simulink library "HighFrequencyNoiseEstimatorCoh"  (R2022b)
settings: Solver=VariableStepAuto  StartTime=0.0  StopTime=10.0  RelTol=1e-3
values from neighbouring files (symbols this model uses):
  NumAAChannels = NumHFRefChannels + 1    [HighFrequencyNoiseEstimatorCohMask.m]
  NumHFRefChannels = NumHFRefLPF + NumHFRefBPF    [HighFrequencyNoiseEstimatorCohMask.m]
undefined symbols (not defined in the file or in its folder): magnitude, Row
libraries: TuneVar x46, TOP x12, StateVar x10, FeaturePath x7, HandyTextFile x4, RfftLib x2, dspmathops x2, dspobslib x2, SpeedBoundsNoiseSlew x2, PooliirLib x2, TSP x1, dspsrcs4 x1
(part 1 of 2)
settings Model: Creator=zs14328  LastModifiedBy=sc48041
settings SolverCC: AlgebraicLoopSolver=TrustRegion
settings DataIOCC: ReturnWorkspaceOutputs=off
settings DebuggingCC: UnconnectedInputMsg=warning  UnconnectedOutputMsg=warning  UnconnectedLineMsg=warning  SFMachineParentedDataDiag=warning  ArithmeticOperatorsInVariantConditions=warning
settings ModelReferenceCC: EnableRefExpFcnMdlSchedulingChecks=on
settings SFSimCC: CustomCodeUndefinedFunction=UseInterfaceOnly

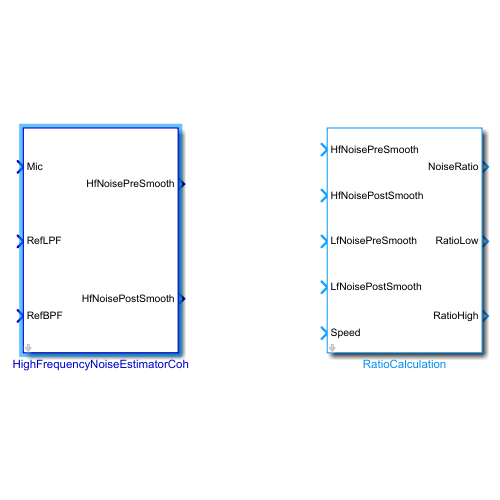
[thumbnail: Simulink's stored preview of the top-level diagram]
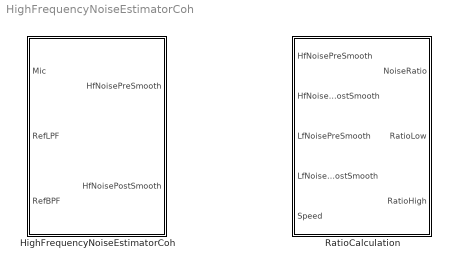
== system HighFrequencyNoiseEstimatorCoh ==
  HighFrequencyNoiseEstimatorCoh : Subsystem  mask(AudioPilot - High-Frequency Noise Estimator){FeatureName=HfNoise, NumHFRefLPF=4, NumHFRefBPF=3, Config=[], TriggerInit=0}
      mask prompts: FeatureName "Feature Name:"; NumHFRefLPF "Number of "High-Pass" Reference Channels"; NumHFRefBPF "Number of "Full-Band" Reference Channels"; Config "HighFrequencyNoiseEstimatorCohConfig"
      mask help: This block implements the high-frequency noise estimator based on the multi-coherence method.
      mask init:
      | blkh = gcbh;
      | 
      | Config = BTConfig.Assert(blkh,Config);
      | Config.Validate();
      | 
      | % Matlab Function Parameters
      | FrameSize = Config.FrameSize;
      | SampleRate = Config.SampleRateHz;
      | HFDecRate = Config.DecRateHz;
      | HFDecRate2 = Config.CoherenceDecRateHz;
      | HFDecRate3 = Config.CoherenceDecRate2Hz;   
      | 
      | % Constants
      | 
      | EmptyStftInput = zeros((FrameSize/Config.DecimationFactor),1);
      |           
      | % Create the PoolIIR Coefficients and Parameters           
      | [AA, BPLP, NumAAChannels, NumHFRefChannels] ...
      |     = HighFrequencyNoiseEstimatorCohMask.FormFilterCoef ...
      |                 (blkh,Config,NumHFRefLPF,NumHFRefBPF);
      | 
      | % Configure Model according to Mask & Config Parameters            
      | HighFrequencyNoiseEstimatorCohMask.ConfigureModel ...
      |                 (blkh,NumHFRefLPF,NumHFRefBPF,Config);
      | 
      | BTConfig.InitSetFeatureIfPresent(blkh,'FeatureName');
      mask Help:
      | Arguments for this block:
      | 
      | Design Time Configuration
      | 
      | Feature Name -
      | The Feature Name can be specified unless a BTC instance is used, in which case, the instance name will be used as Feature Name.
      | 
      | Number of "High-Pass"Reference Channels -
      | These are the reference channels from Medusa that have already been high-passed, such as  Limp, Rimp etc.  These channels will then undergo low-pass filtering only.
      | 
      | Number of "Full-Band" Reference Channels -
      | These are the reference channels from Medusa that are essentially full-band, such as LStreb, RStreb etc.  These channels will then undergo band-pass filtering.
      | 
      | Build Time Configuration -
      | The block can be configured using a object of class, HighFrequencyNoiseEstimatorCohConfig.
      mask TypeOptions FeatureName: FeaturePath/FeatureName
      mask Callback Config: BTConfig.CallbackHideIfPresent(gcbh,{'FeatureName'});
      mask Callback TriggerInit: HighFrequencyNoiseEstimatorCohMask.TriggerInitCallBack(gcbh);
      mask DialogControl DTCTitle Prompt: <b>Design Time Configuration</b>
      mask DialogControl BTCTitle Prompt: <b>Build Time Configuration</b>
  RatioCalculation : Subsystem  mask(AudioPilot - Noise Ratio Calculation){FeatureName=Ratio, Config=[]}
      mask prompts: FeatureName "Feature Name:"; Config "RatioCalculationConfig"
      mask help: This block handles the computation, smoothing and impulse rejection of the noise ratio.
      mask init:
      | blkh = gcbh;
      | 
      | Config = BTConfig.Assert(blkh,Config);
      | Config.Validate();
      | 
      | SampleRate = Config.SampleRateHz;
      | HFDecRate = Config.DecRateHz;
      |  
      | BTConfig.InitSetFeatureIfPresent(blkh,'FeatureName');
      mask Help:
      | This block handles the computation, smoothing and impulse rejection of the noise ratio.
      | 
      | Arguments for this block:
      | 
      | Design Time Configuration
      | The Feature Name can be specified unless a BTC instance is used, in which case, the instance name will be used as Feature Name.
      | 
      | Build Time Configuration
      | The block can be configured using a object of class, RatioCalculationConfig.
      mask TypeOptions FeatureName: FeaturePath/FeatureName
      mask Callback Config: BTConfig.CallbackHideIfPresent(gcbh,{'FeatureName'});
      mask DialogControl DTCTitle Prompt: <b>Design Time Configuration </b>
      mask DialogControl BTCTitle Prompt: <b>Build Time Configuration </b>
      mask DialogControl Config Tooltip: The configuration has to be an object of the class, RatioCalculationConfig.

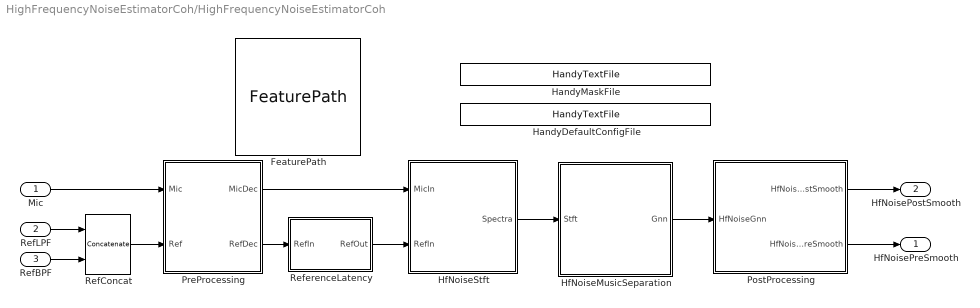
== system HighFrequencyNoiseEstimatorCoh/HighFrequencyNoiseEstimatorCoh ==
  Mic : Inport
  RefLPF : Inport  Port=2  PortDimensions=[FrameSize NumHFRefLPF]
  RefBPF : Inport  Port=3  PortDimensions=[FrameSize NumHFRefBPF]
  FeaturePath : FeaturePath/FeaturePath  FeatureName=HfNoise  IsGroup=off  GroupNumber=-1  IsModule=off  TriggerInit=[360 -186 485 -69]
      settings: SourceProductName=Bose Talaria
  HandyDefaultConfigFile : HandyTextFile/HandyTextFile  TemplateSource=Config  FileSuffix=Init  OpenDialogOnLoad=off  UseThisBlockName=off  AddGrandParentNamePrefix=off  TheDefaultText=|  ShowInLibBrowser=on
      | % $(FILENAME) Setup model parameters for each "Init" callback (e.g. update diagram)
      | sample_rate_in_hertz = 44100;
      | frame_size = 32;
      | sysin_channel_count = 2;
      settings: SourceProductName=Bose Talaria
  HandyMaskFile : HandyTextFile/HandyTextFile  TemplateSource=<dialog fields>  FileSuffix=Mask  OpenDialogOnLoad=off  UseThisBlockName=off  AddGrandParentNamePrefix=off  TheDefaultText=|  ShowInLibBrowser=on
      | % $(FILENAME) Setup model parameters for each "Init" callback (e.g. update diagram)
      | sample_rate_in_hertz = 44100;
      | frame_size = 32;
      | sysin_channel_count = 2;
      settings: SourceProductName=Bose Talaria
  "HfNoiseMusicSeparation " : Subsystem
  HfNoiseStft : Subsystem  Variant=on  VariantControlMode=label  LabelModeActiveChoice=EvenNumChannels
  PostProcessing : Subsystem
  PreProcessing : Subsystem
  RefConcat : Concatenate  Mode=Multidimensional array  ConcatenateDimension=2
  ReferenceLatency : Subsystem
  HfNoisePreSmooth : Outport  VectorParamsAs1DForOutWhenUnconnected=off
  HfNoisePostSmooth : Outport  Port=2  VectorParamsAs1DForOutWhenUnconnected=off
  wires:
  "HfNoiseMusicSeparation "/1(Gnn) -> PostProcessing/1(HfNoiseGnn)
  PreProcessing/2(RefDec) -> ReferenceLatency/1(RefIn)
  PreProcessing/1(MicDec) -> HfNoiseStft/1(MicIn)
  PostProcessing/2(HfNoisePreSmooth) -> HfNoisePreSmooth/1
  PostProcessing/1(HfNoisePostSmooth) -> HfNoisePostSmooth/1
  Mic/1 -> PreProcessing/1(Mic)
  HfNoiseStft/1(Spectra) -> "HfNoiseMusicSeparation "/1(Stft)
  ReferenceLatency/1(RefOut) -> HfNoiseStft/2(RefIn)
  RefConcat/1 -> PreProcessing/2(Ref)
  RefLPF/1 -> RefConcat/1
  RefBPF/1 -> RefConcat/2

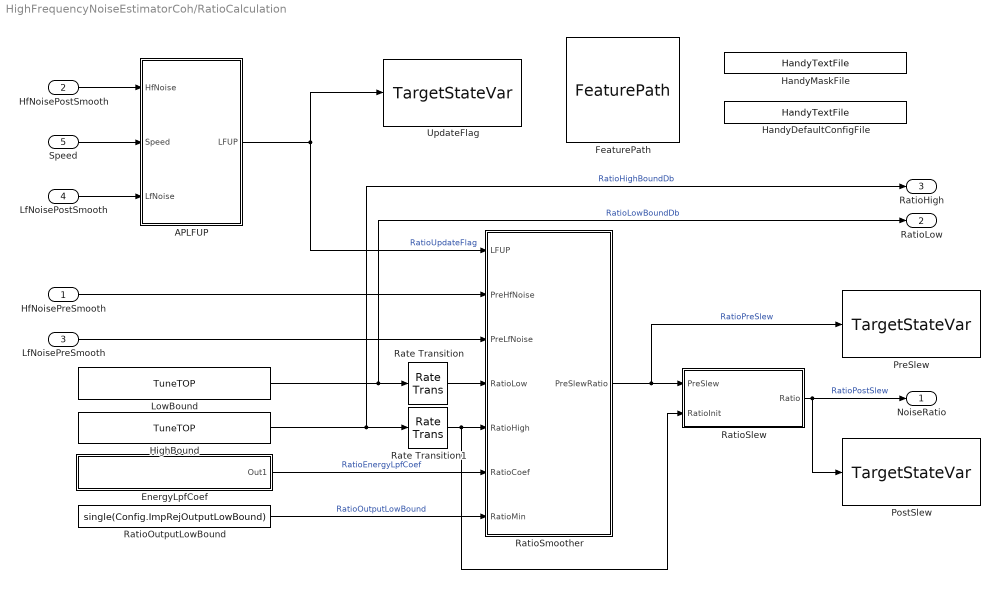
== system HighFrequencyNoiseEstimatorCoh/RatioCalculation ==
  HfNoisePreSmooth : Inport  SampleTime=Config.DecSampleTimeSec
  HfNoisePostSmooth : Inport  Port=2  SampleTime=Config.DecSampleTimeSec
  LfNoisePreSmooth : Inport  Port=3  SampleTime=Config.DecSampleTimeSec
  LfNoisePostSmooth : Inport  Port=4  SampleTime=Config.DecSampleTimeSec
  Speed : Inport  Port=5  SampleTime=Config.DecSampleTimeSec
  APLFUP : Subsystem
  EnergyLpfCoef : Subsystem
  FeaturePath : FeaturePath/FeaturePath  FeatureName=Ratio  IsGroup=off  GroupNumber=-1  IsModule=off  TriggerInit=[735 -166 850 -59]
      settings: SourceProductName=Bose Talaria
  HandyDefaultConfigFile : HandyTextFile/HandyTextFile  TemplateSource=Config  FileSuffix=Init  OpenDialogOnLoad=off  UseThisBlockName=off  TheDefaultText=|  ShowInLibBrowser=on
      | % $(FILENAME) Setup model parameters for each "Init" callback (e.g. update diagram)
      | sample_rate_in_hertz = 44100;
      | frame_size = 32;
      | sysin_channel_count = 2;
      settings: SourceProductName=Bose Talaria
  HandyMaskFile : HandyTextFile/HandyTextFile  TemplateSource=Mask  FileSuffix=Init  OpenDialogOnLoad=off  UseThisBlockName=off  TheDefaultText=|  ShowInLibBrowser=on
      | % $(FILENAME) Setup model parameters for each "Init" callback (e.g. update diagram)
      | sample_rate_in_hertz = 44100;
      | frame_size = 32;
      | sysin_channel_count = 2;
      settings: SourceProductName=Bose Talaria
  HighBound : TuneVar/TuneTOP  TriggerInit=[240 214 435 246]  TopName=HighBoundDb  TuneName=HighBoundDb  DataType=single  TunabilityNumber=1  MinValue=[]  MaxValue=[]  BankNumber=0  PreOverlay=false  PostOverlay=false  UseSameName=on  MaskValue=Config.HighBoundDb
      settings: SourceProductName=Bose Talaria
  LowBound : TuneVar/TuneTOP  TriggerInit=[240 169 435 201]  TopName=LowBoundDb  TuneName=LowBoundDb  DataType=single  TunabilityNumber=1  MinValue=[]  MaxValue=[]  BankNumber=0  PreOverlay=false  PostOverlay=false  UseSameName=on  MaskValue=Config.LowBoundDb
      settings: SourceProductName=Bose Talaria
  PostSlew : StateVar/TargetStateVar  TriggerInit=[1015 241 1155 309]  TspName=PostSlew  StateName=PostSlew  UseSameName=on  IfdefMacro=[]
      settings: SourceProductName=Bose Talaria
  PreSlew : StateVar/TargetStateVar  TriggerInit=[1015 91 1155 159]  TspName=PreSlew  StateName=PreSlew  UseSameName=on  IfdefMacro=[]
      settings: SourceProductName=Bose Talaria
  Rate Transition : RateTransition
  Rate Transition1 : RateTransition
  RatioOutputLowBound : Constant  Value=single(Config.ImpRejOutputLowBound)
  RatioSlew : Subsystem
  RatioSmoother : Subsystem
  UpdateFlag : StateVar/TargetStateVar  TriggerInit=[550 -144 690 -76]  TspName=UpdateFlag  StateName=UpdateFlag  UseSameName=on  IfdefMacro=[]
      settings: SourceProductName=Bose Talaria
  NoiseRatio : Outport  VectorParamsAs1DForOutWhenUnconnected=off
  RatioLow : Outport  Port=2  VectorParamsAs1DForOutWhenUnconnected=off
  RatioHigh : Outport  Port=3  VectorParamsAs1DForOutWhenUnconnected=off
  wires:
  APLFUP/1(LFUP) -> RatioSmoother/1(LFUP), UpdateFlag/1  "RatioUpdateFlag"
  RatioSmoother/1(PreSlewRatio) -> PreSlew/1, RatioSlew/1(PreSlew)  "RatioPreSlew"
  HfNoisePostSmooth/1 -> APLFUP/1(HfNoise)
  RatioSlew/1(Ratio) -> NoiseRatio/1, PostSlew/1  "RatioPostSlew"
  HfNoisePreSmooth/1 -> RatioSmoother/2(PreHfNoise)
  EnergyLpfCoef/1(Out1) -> RatioSmoother/6(RatioCoef)  "RatioEnergyLpfCoef"
  RatioOutputLowBound/1 -> RatioSmoother/7(RatioMin)  "RatioOutputLowBound"
  HighBound/1 -> RatioHigh/1, Rate Transition1/1  "RatioHighBoundDb"
  LowBound/1 -> RatioLow/1, Rate Transition/1  "RatioLowBoundDb"
  Speed/1 -> APLFUP/2(Speed)
  LfNoisePostSmooth/1 -> APLFUP/3(LfNoise)
  LfNoisePreSmooth/1 -> RatioSmoother/3(PreLfNoise)
  Rate Transition/1 -> RatioSmoother/4(RatioLow)
  Rate Transition1/1 -> RatioSlew/2(RatioInit), RatioSmoother/5(RatioHigh)

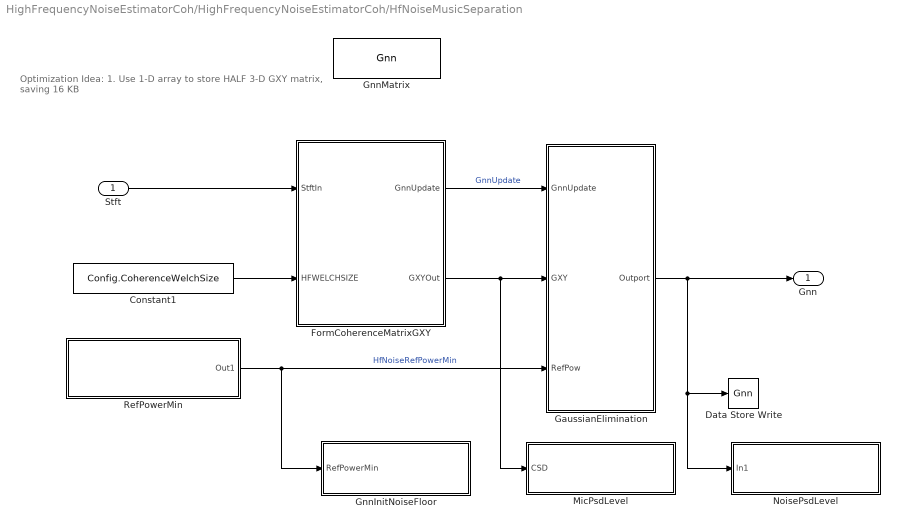
== system HighFrequencyNoiseEstimatorCoh/HighFrequencyNoiseEstimatorCoh/HfNoiseMusicSeparation  ==
  note: Optimization Idea:
      | 1. Use 1-D array to store HALF 3-D GXY matrix, saving 16 KB
  Stft : Inport
  Constant1 : Constant  Value=Config.CoherenceWelchSize  OutDataTypeStr=single
  Data Store Write : DataStoreWrite  DataStoreName=Gnn  IndexOptions=Index vector (dialog)  Indices=1  OutputSizes=1
  FormCoherenceMatrixGXY : MATLAB Function  TreatAsAtomicUnit=on
  GaussianElimination : Subsystem
  GnnInitNoiseFloor : MATLAB Function  TreatAsAtomicUnit=on
  GnnMatrix : DataStoreMemory  DataStoreName=Gnn  InitialValue=single(zeros(Config.CoherenceFftSize/4+1,1))  ShowAdditionalParam=off  OutDataTypeStr=single
  MicPsdLevel : Subsystem
  NoisePsdLevel : Subsystem
  RefPowerMin : Subsystem
  Gnn : Outport  VectorParamsAs1DForOutWhenUnconnected=off
  wires:
  RefPowerMin/1(Out1) -> GnnInitNoiseFloor/1(RefPowerMin), GaussianElimination/3(RefPow)  "HfNoiseRefPowerMin"
  FormCoherenceMatrixGXY/2(GXYOut) -> MicPsdLevel/1(CSD), GaussianElimination/2(GXY)
  FormCoherenceMatrixGXY/1(GnnUpdate) -> GaussianElimination/1(GnnUpdate)  "GnnUpdate"
  GaussianElimination/1(Outport) -> NoisePsdLevel/1(In1), Data Store Write/1, Gnn/1
  Constant1/1 -> FormCoherenceMatrixGXY/2(HFWELCHSIZE)
  Stft/1 -> FormCoherenceMatrixGXY/1(StftIn)

== system HighFrequencyNoiseEstimatorCoh/HighFrequencyNoiseEstimatorCoh/HfNoiseStft ==
  MicIn : Inport
  RefIn : Inport  Port=2
  EvenNumChannels : Subsystem  VariantControl=EvenNumChannels
  OddNumChannels : Subsystem  VariantControl=OddNumChannels
  Spectra : Outport

== system HighFrequencyNoiseEstimatorCoh/HighFrequencyNoiseEstimatorCoh/PostProcessing ==
  HfNoiseGnn : Inport  SampleTime=1/HFDecRate2
  HfImpulseRejection : Subsystem
  HfSlew : Subsystem
  PostSlew : StateVar/TargetStateVar  TriggerInit=[735 161 875 229]  TspName=PostSlew  StateName=PostSlew  UseSameName=on  IfdefMacro=[]
      settings: SourceProductName=Bose Talaria
  PreSlew : StateVar/TargetStateVar  TriggerInit=[735 251 875 319]  TspName=PreSlew  StateName=PreSlew  UseSameName=on  IfdefMacro=[]
      settings: SourceProductName=Bose Talaria
  offset : TuneVar/TuneTOP  TriggerInit=[-35 192 190 228]  TopName=OffsetDb  TuneName=OffsetDb  DataType=single  TunabilityNumber=1  MinValue=[]  MaxValue=[]  BankNumber=0  PreOverlay=false  PostOverlay=false  UseSameName=on  MaskValue=Config.NoiseLevelBias
      settings: SourceProductName=Bose Talaria
  HfNoisePostSmooth : Outport  VectorParamsAs1DForOutWhenUnconnected=off
  HfNoisePreSmooth : Outport  Port=2  VectorParamsAs1DForOutWhenUnconnected=off
  wires:
  HfImpulseRejection/1(HfNoisePreSlew) -> PreSlew/1, HfNoisePreSmooth/1, HfSlew/1(HfNoisePreSlew)  "HfNoisePreSlew"
  HfSlew/1(HfNoisePostSlew) -> PostSlew/1, HfNoisePostSmooth/1  "HfNoisePostSlew"
  HfNoiseGnn/1 -> HfImpulseRejection/1(HfPowSpecDec)
  offset/1 -> HfImpulseRejection/2(LevelOffset)  "HfNoiseOffsetDb"

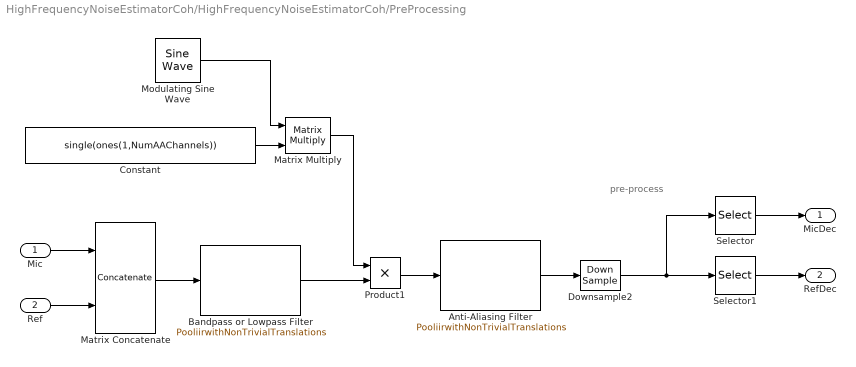
== system HighFrequencyNoiseEstimatorCoh/HighFrequencyNoiseEstimatorCoh/PreProcessing ==
  note: pre-process
  Mic : Inport
  Ref : Inport  Port=2
  Anti-Aliasing Filter : PooliirLib/PooliirwithNonTrivialTranslations  maxNumStages=AA.MaxNumStages  numStages=AA.NumStages  sosCoefficients=AA.SOS  alias='HFAA'  variantType=Config.AaFiltVariant  FeatureName=PreprocessAntiAlias
  Bandpass or Lowpass Filter : PooliirLib/PooliirwithNonTrivialTranslations  maxNumStages=BPLP.MaxNumStages  numStages=BPLP.NumStages  sosCoefficients=BPLP.SOS  alias='HFBPFilt'  variantType=Config.BpLpFiltVariant  FeatureName=PreprocessBandpassLowpass
  Constant : Constant  Value=single(ones(1,NumAAChannels))  VectorParams1D=off
  Downsample2 : DownSample  N=Config.DecimationFactor
  Matrix Concatenate : Concatenate  Mode=Multidimensional array  ConcatenateDimension=2
  Matrix Multiply : Product  Multiplication=Matrix(*)
  Modulating Sine Wave : dspsrcs4/Sine Wave  Amplitude=1  Frequency=Config.ModulateFrequencyHz  Phase=0  SampleMode=Discrete  OutComplex=Real  CompMethod=Table lookup  TableSize=Speed  SampleTime=1/SampleRate  SamplesPerFrame=FrameSize  ResetState=Restart at time zero  OutputFrames=off  dataType=single  wordLen=16  udDataType=sfix(16)  fracBitsMode=Best precision  numFracBits=15  OutDataTypeStr=single  LastOutDataTypeStr=single
  Product1 : Product  RndMeth=Zero
  Selector : Selector  NumberOfDimensions=2  InputPortWidth=3  IndexOptions=Select all,Index vector (dialog)  Indices=[1 3],1  OutputSizes=1,1
  Selector1 : Selector  NumberOfDimensions=2  InputPortWidth=3  IndexOptions=Select all,Starting index (dialog)  Indices=[1 3],2  OutputSizes=1,NumHFRefChannels
  MicDec : Outport  VectorParamsAs1DForOutWhenUnconnected=off
  RefDec : Outport  Port=2  VectorParamsAs1DForOutWhenUnconnected=off
  wires:
  Matrix Multiply/1 -> Product1/1
  Constant/1 -> Matrix Multiply/2
  Anti-Aliasing Filter/1 -> Downsample2/1
  Mic/1 -> Matrix Concatenate/1
  Bandpass or Lowpass Filter/1 -> Product1/2
  Product1/1 -> Anti-Aliasing Filter/1
  Downsample2/1 -> Selector/1, Selector1/1
  Ref/1 -> Matrix Concatenate/2
  Matrix Concatenate/1 -> Bandpass or Lowpass Filter/1
  Selector/1 -> MicDec/1
  Selector1/1 -> RefDec/1
  Modulating Sine Wave/1 -> Matrix Multiply/1

== system HighFrequencyNoiseEstimatorCoh/HighFrequencyNoiseEstimatorCoh/ReferenceLatency ==
  RefIn : Inport
  Delay : TunableDelay/Delay  maxDelayTime=Config.RefMaxLatencySamples  frameSize=FrameSize/Config.DecimationFactor  numChannels=NumHFRefChannels  bufferAlias=[]  headerFilename=[]
  RefLatency : Subsystem
  RefOut : Outport  VectorParamsAs1DForOutWhenUnconnected=off
  wires:
  Delay/1 -> RefOut/1
  RefIn/1 -> Delay/1
  RefLatency/1(hf_noise_ref_latency_samples) -> Delay/2  "hf_noise_ref_latency_samples"

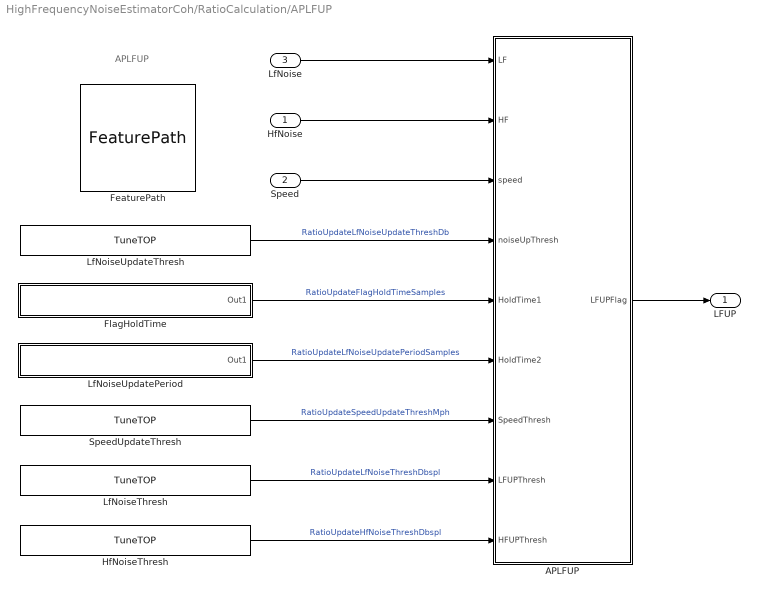
== system HighFrequencyNoiseEstimatorCoh/RatioCalculation/APLFUP ==
  note: APLFUP
  HfNoise : Inport
  Speed : Inport  Port=2
  LfNoise : Inport  Port=3
  APLFUP : MATLAB Function  TreatAsAtomicUnit=on
  FeaturePath : FeaturePath/FeaturePath  FeatureName=Update  IsGroup=off  GroupNumber=-1  IsModule=off  TriggerInit=[-40 39 75 146]
      settings: SourceProductName=Bose Talaria
  FlagHoldTime : Subsystem
  HfNoiseThresh : TuneVar/TuneTOP  TriggerInit=[-100 480 130 510]  TopName=HfNoiseThreshDbspl  TuneName=HfNoiseThreshDbspl  DataType=single  TunabilityNumber=1  MinValue=[]  MaxValue=[]  BankNumber=0  PreOverlay=false  PostOverlay=false  UseSameName=on  MaskValue=Config.UpdateHfNoiseThreshDbspl
      settings: SourceProductName=Bose Talaria
  LfNoiseThresh : TuneVar/TuneTOP  TriggerInit=[-100 420 130 450]  TopName=LfNoiseThreshDbspl  TuneName=LfNoiseThreshDbspl  DataType=single  TunabilityNumber=1  MinValue=[]  MaxValue=[]  BankNumber=0  PreOverlay=false  PostOverlay=false  UseSameName=on  MaskValue=Config.UpdateLfNoiseThreshDbspl
      settings: SourceProductName=Bose Talaria
  LfNoiseUpdatePeriod : Subsystem
  LfNoiseUpdateThresh : TuneVar/TuneTOP  TriggerInit=[-100 180 130 210]  TopName=LfNoiseUpdateThreshDb  TuneName=LfNoiseUpdateThreshDb  DataType=single  TunabilityNumber=1  MinValue=[]  MaxValue=[]  BankNumber=0  PreOverlay=false  PostOverlay=false  UseSameName=on  MaskValue=Config.UpdateLfNoiseUpdateThreshDb
      settings: SourceProductName=Bose Talaria
  SpeedUpdateThresh : TuneVar/TuneTOP  TriggerInit=[-100 360 130 390]  TopName=SpeedUpdateThreshMph  TuneName=SpeedUpdateThreshMph  DataType=single  TunabilityNumber=1  MinValue=[]  MaxValue=[]  BankNumber=0  PreOverlay=false  PostOverlay=false  UseSameName=on  MaskValue=Config.UpdateSpeedUpdateThreshMph
      settings: SourceProductName=Bose Talaria
  LFUP : Outport  VectorParamsAs1DForOutWhenUnconnected=off
  wires:
  LfNoise/1 -> APLFUP/1(LF)
  HfNoise/1 -> APLFUP/2(HF)
  Speed/1 -> APLFUP/3(speed)
  APLFUP/1(LFUPFlag) -> LFUP/1
  HfNoiseThresh/1 -> APLFUP/9(HFUPThresh)  "RatioUpdateHfNoiseThreshDbspl"
  LfNoiseUpdateThresh/1 -> APLFUP/4(noiseUpThresh)  "RatioUpdateLfNoiseUpdateThreshDb"
  LfNoiseUpdatePeriod/1(Out1) -> APLFUP/6(HoldTime2)  "RatioUpdateLfNoiseUpdatePeriodSamples"
  SpeedUpdateThresh/1 -> APLFUP/7(SpeedThresh)  "RatioUpdateSpeedUpdateThreshMph"
  LfNoiseThresh/1 -> APLFUP/8(LFUPThresh)  "RatioUpdateLfNoiseThreshDbspl"
  FlagHoldTime/1(Out1) -> APLFUP/5(HoldTime1)  "RatioUpdateFlagHoldTimeSamples"

== system HighFrequencyNoiseEstimatorCoh/RatioCalculation/EnergyLpfCoef ==
  TOP : TOP/TOP  TriggerInit=[220 20 470 80]  TopName=EnergyLpfCoef  DataType=single  BankNumber=0  PreOverlay=false  PostOverlay=false  Role=Automatic
      settings: SourceProductName=Bose Talaria
  Tau2Coef : MATLAB Function  TreatAsAtomicUnit=on
  TranslateTrigger : TuneVar/TranslateTrigger  TriggerInit=[96 -105 134 -50]
      settings: SourceProductName=Bose Talaria
  Tune Variable : TuneVar/TuneVar  TuneName=EnergyLpfTauS  SpecifyMaxSize=off  VariableDim=1 (Row)  MaxSize=[1 1]  TunabilityNumber=1  MinValue=[]  MaxValue=[]  TriggerInit=[-315 20 -65 80]  MaskValue=Config.ImpRejEnergyLpfTauSec
      settings: SourceProductName=Bose Talaria
  Out1 : Outport  VectorParamsAs1DForOutWhenUnconnected=off
  wires:
  TOP/1 -> Out1/1  "EnergyLpfCoef"
  Tune Variable/1 -> Tau2Coef/1(tau)  "EnergyLpfTauS"
  Tau2Coef/1(coef) -> TOP/1
  TranslateTrigger/1 -> Tau2Coef/Trigger

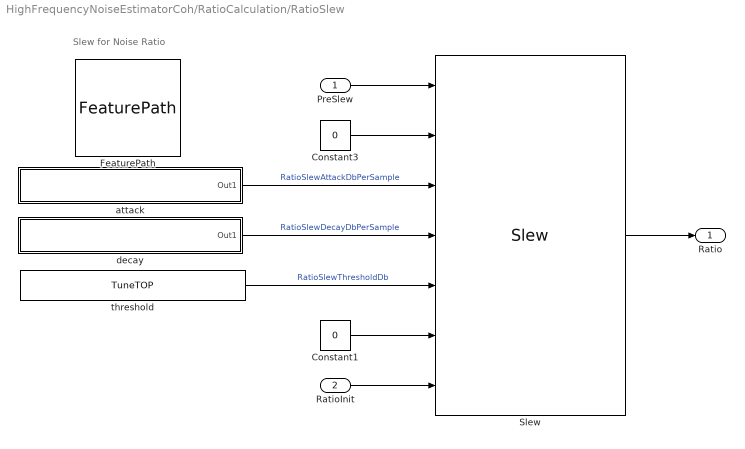
== system HighFrequencyNoiseEstimatorCoh/RatioCalculation/RatioSlew ==
  note: Slew for Noise Ratio
  PreSlew : Inport
  RatioInit : Inport  Port=2
  Constant1 : Constant  Value=0  OutDataTypeStr=single
  Constant3 : Constant  Value=0  OutDataTypeStr=single
  FeaturePath : FeaturePath/FeaturePath  FeatureName=Slew  IsGroup=off  GroupNumber=-1  IsModule=off  TriggerInit=[-130 34 -25 131]
      settings: SourceProductName=Bose Talaria
  Slew : SpeedBoundsNoiseSlew/Slew  SystemSampleTime=-1  VariantActivationTime=update diagram  Latency=0  AutoFrameSizeCalculation=off
  attack : Subsystem
  decay : Subsystem
  threshold : TuneVar/TuneTOP  TriggerInit=[-185 245 40 275]  TopName=ThresholdDb  TuneName=ThresholdDb  DataType=single  TunabilityNumber=1  MinValue=[]  MaxValue=[]  BankNumber=0  PreOverlay=false  PostOverlay=false  UseSameName=on  MaskValue=Config.SlewThresholdDb
      settings: SourceProductName=Bose Talaria
  Ratio : Outport  VectorParamsAs1DForOutWhenUnconnected=off
  wires:
  Slew/1 -> Ratio/1
  PreSlew/1 -> Slew/1
  Constant3/1 -> Slew/2
  decay/1(Out1) -> Slew/4  "RatioSlewDecayDbPerSample"
  threshold/1 -> Slew/5  "RatioSlewThresholdDb"
  attack/1(Out1) -> Slew/3  "RatioSlewAttackDbPerSample"
  RatioInit/1 -> Slew/7
  Constant1/1 -> Slew/6

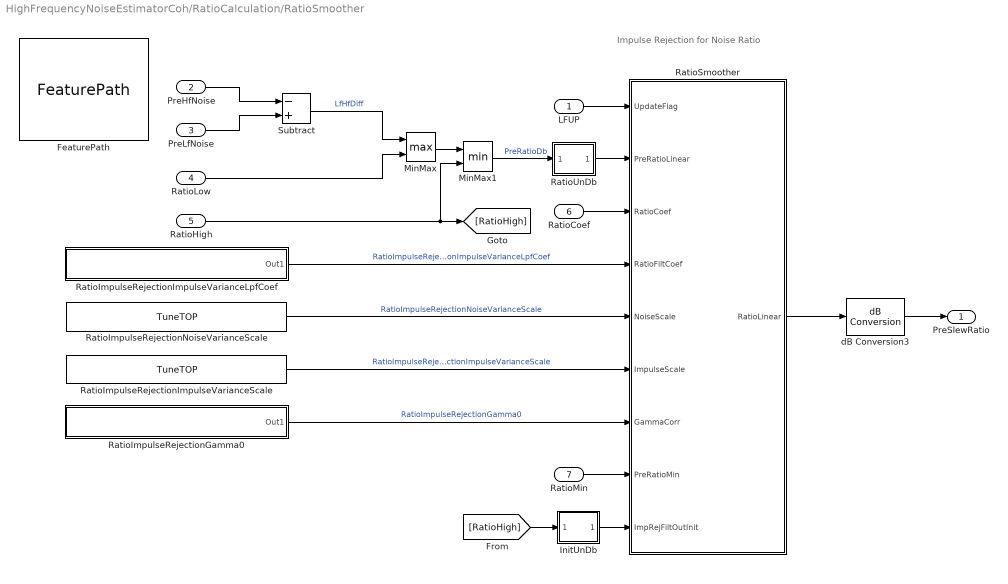
== system HighFrequencyNoiseEstimatorCoh/RatioCalculation/RatioSmoother ==
  note: Impulse Rejection for Noise Ratio
  LFUP : Inport  SampleTime=Config.DecSampleTimeSec
  PreHfNoise : Inport  Port=2  SampleTime=Config.DecSampleTimeSec
  PreLfNoise : Inport  Port=3  SampleTime=Config.DecSampleTimeSec
  RatioLow : Inport  Port=4  SampleTime=Config.DecSampleTimeSec
  RatioHigh : Inport  Port=5  SampleTime=Config.DecSampleTimeSec
  RatioCoef : Inport  Port=6  SampleTime=Config.DecSampleTimeSec
  RatioMin : Inport  Port=7  SampleTime=Config.DecSampleTimeSec
  FeaturePath : FeaturePath/FeaturePath  FeatureName=ImpulseRejection  IsGroup=off  GroupNumber=-1  IsModule=off  TriggerInit=[-30 114 105 221]
      settings: SourceProductName=Bose Talaria
  InitUnDb : Subsystem  mask(dB Deconversion){}
      mask help: This block converts dB to amplitude.
  MinMax : MinMax  Function=max  Inputs=2
  MinMax1 : MinMax  Inputs=2  OutDataTypeStr=single
  RatioImpulseRejectionGamma0 : Subsystem
  RatioImpulseRejectionImpulseVarianceLpfCoef : Subsystem
  RatioImpulseRejectionImpulseVarianceScale : TuneVar/TuneTOP  TriggerInit=[20 445 250 475]  TopName=ImpulseVarianceScale  TuneName=ImpulseVarianceScale  DataType=single  TunabilityNumber=1  MinValue=[]  MaxValue=[]  BankNumber=0  PreOverlay=false  PostOverlay=false  UseSameName=on  MaskValue=Config.ImpRejImpulseScale
      settings: SourceProductName=Bose Talaria
  RatioImpulseRejectionNoiseVarianceScale : TuneVar/TuneTOP  TriggerInit=[20 390 250 420]  TopName=NoiseVarianceScale  TuneName=NoiseVarianceScale  DataType=single  TunabilityNumber=1  MinValue=[]  MaxValue=[]  BankNumber=0  PreOverlay=false  PostOverlay=false  UseSameName=on  MaskValue=Config.ImpRejNoiseScale
      settings: SourceProductName=Bose Talaria
  RatioSmoother : MATLAB Function  TreatAsAtomicUnit=on
  RatioUnDb : Subsystem  mask(dB Deconversion){}
      mask help: This block converts dB to amplitude.
  Subtract : Sum  Inputs=-+
  dB Conversion3 : dspmathops/dB Conversion  dBtype=dB  intype=Amplitude  R=1  fuzz=on
  PreSlewRatio : Outport  VectorParamsAs1DForOutWhenUnconnected=off
  wires:
  PreLfNoise/1 -> Subtract/2
  dB Conversion3/1 -> PreSlewRatio/1
  Subtract/1 -> MinMax/1  "LfHfDiff"
  RatioSmoother/1(RatioLinear) -> dB Conversion3/1
  MinMax1/1 -> RatioUnDb/1(" ")  "PreRatioDb"
  MinMax/1 -> MinMax1/1
  PreHfNoise/1 -> Subtract/1
  LFUP/1 -> RatioSmoother/1(UpdateFlag)
  RatioUnDb/1("  ") -> RatioSmoother/2(PreRatioLinear)
  RatioHigh/1 -> [RatioHigh], MinMax1/2
  RatioLow/1 -> MinMax/2
  RatioCoef/1 -> RatioSmoother/3(RatioCoef)
  RatioMin/1 -> RatioSmoother/8(PreRatioMin)
  RatioImpulseRejectionImpulseVarianceLpfCoef/1(Out1) -> RatioSmoother/4(RatioFiltCoef)  "RatioImpulseRejectionImpulseVarianceLpfCoef"
  RatioImpulseRejectionNoiseVarianceScale/1 -> RatioSmoother/5(NoiseScale)  "RatioImpulseRejectionNoiseVarianceScale"
  RatioImpulseRejectionImpulseVarianceScale/1 -> RatioSmoother/6(ImpulseScale)  "RatioImpulseRejectionImpulseVarianceScale"
  RatioImpulseRejectionGamma0/1(Out1) -> RatioSmoother/7(GammaCorr)  "RatioImpulseRejectionGamma0"
  InitUnDb/1("  ") -> RatioSmoother/9(ImpRejFiltOutInit)
  [RatioHigh] -> InitUnDb/1(" ")

== system HighFrequencyNoiseEstimatorCoh/HighFrequencyNoiseEstimatorCoh/HfNoiseMusicSeparation /GaussianElimination ==
  GnnUpdate : Inport
  GXY : Inport  Port=2
  RefPow : Inport  Port=3
  Data Store Read1 : DataStoreRead  DataStoreName=Gnn  IndexOptions=Index vector (dialog)  Indices=1  OutputSizes=1
  If : If  IfExpression=u1
  If Action Subsystem : Subsystem  TreatAsAtomicUnit=on
  If Action Subsystem1 : Subsystem  TreatAsAtomicUnit=on
  Merge : Merge
  Outport : Outport  VectorParamsAs1DForOutWhenUnconnected=off
  wires:
  GXY/1 -> If Action Subsystem/2(GXY)
  Merge/1 -> Outport/1
  RefPow/1 -> If Action Subsystem/1(RefPowMin)  "HFNoiseRefPowerMin"
  Data Store Read1/1 -> If Action Subsystem1/1(Gnn)
  GnnUpdate/1 -> If/1
  If Action Subsystem/1(Out1) -> Merge/2
  If/2 -> If Action Subsystem1/Action
  If Action Subsystem1/1(Out1) -> Merge/1
  If/1 -> If Action Subsystem/Action

== system HighFrequencyNoiseEstimatorCoh/HighFrequencyNoiseEstimatorCoh/HfNoiseMusicSeparation /MicPsdLevel ==
  CSD : Inport
  ExtractMicLevel : MATLAB Function  TreatAsAtomicUnit=on
  TargetStateVar : StateVar/TargetStateVar  TriggerInit=[-280 -89 -140 -21]  TspName=MicPsdLevel  StateName=MicPsdLevel  UseSameName=on  IfdefMacro=[]
      settings: SourceProductName=Bose Talaria
  wires:
  CSD/1 -> ExtractMicLevel/1(CSD)
  ExtractMicLevel/1(MicLevel) -> TargetStateVar/1

== system HighFrequencyNoiseEstimatorCoh/HighFrequencyNoiseEstimatorCoh/HfNoiseMusicSeparation /NoisePsdLevel ==
  In1 : Inport
  ExtractNoiseLevel : MATLAB Function  TreatAsAtomicUnit=on  mask(Talaria Interpretation){}
      mask help: This MATLAB Function Block can be automatically inserted by several automation routines. Once placed, the block is ready to accept interpretation logic from the model designer.
  InterpretTrigger : StateVar/InterpretTrigger  TriggerInit=[331 20 369 75]
      settings: SourceProductName=Bose Talaria
  StateVar : StateVar/StateVar  TriggerInit=[490 139 605 201]  StateName=NoisePsdLevel
      settings: SourceProductName=Bose Talaria
  TSP : TSP/TSP  TriggerInit=[110 138 270 202]  TspName=PowerSpectralDensity  IfDefMacro=[]  Role=Automatic
      settings: SourceProductName=Bose Talaria
  wires:
  In1/1 -> TSP/1
  TSP/1 -> ExtractNoiseLevel/1(PSD)
  InterpretTrigger/1 -> ExtractNoiseLevel/Trigger
  ExtractNoiseLevel/1(NoiseLevel) -> StateVar/1

== system HighFrequencyNoiseEstimatorCoh/HighFrequencyNoiseEstimatorCoh/HfNoiseMusicSeparation /RefPowerMin ==
  RefPowerMin : TOP/TOP  TriggerInit=[440 20 585 80]  TopName=RefPowerMin  DataType=single  BankNumber=0  PreOverlay=false  PostOverlay=false  Role=Automatic
      settings: SourceProductName=Bose Talaria
  TranslateTrigger : TuneVar/TranslateTrigger  TriggerInit=[306 -100 344 -45]
      settings: SourceProductName=Bose Talaria
  Tune Variable : TuneVar/TuneVar  TuneName=RefPowerMinDb  SpecifyMaxSize=off  VariableDim=1 (Row)  MaxSize=[1 1]  TunabilityNumber=1  MinValue=[]  MaxValue=[]  TriggerInit=[-25 25 145 75]  MaskValue=Config.RefPowerMinDb
      settings: SourceProductName=Bose Talaria
  undB : MATLAB Function  TreatAsAtomicUnit=on
  Out1 : Outport  VectorParamsAs1DForOutWhenUnconnected=off
  wires:
  RefPowerMin/1 -> Out1/1  "RefPowerMin"
  Tune Variable/1 -> undB/1(Tune)  "RefPowerMinDb"
  undB/1(TOP) -> RefPowerMin/1
  TranslateTrigger/1 -> undB/Trigger

== system HighFrequencyNoiseEstimatorCoh/HighFrequencyNoiseEstimatorCoh/HfNoiseStft/EvenNumChannels ==
  MicIn : Inport
  RefIn : Inport  Port=2
  Matrix Concatenate : Concatenate  Mode=Multidimensional array  ConcatenateDimension=2
  "StftRef " : Subsystem
  Spectra : Outport
  wires:
  MicIn/1 -> Matrix Concatenate/2
  RefIn/1 -> Matrix Concatenate/1
  "StftRef "/1(StftOut) -> Spectra/1
  Matrix Concatenate/1 -> "StftRef "/1(data)

== system HighFrequencyNoiseEstimatorCoh/HighFrequencyNoiseEstimatorCoh/HfNoiseStft/OddNumChannels ==
  MicIn : Inport
  RefIn : Inport  Port=2
  Constant : Constant  Value=EmptyStftInput  VectorParams1D=off  OutDataTypeStr=single
  Matrix Concatenate : Concatenate  NumInputs=3  Mode=Multidimensional array  ConcatenateDimension=2
  Selector : Selector  NumberOfDimensions=2  InputPortWidth=3  IndexOptions=Select all,Index vector (dialog)  Indices=[1 3],[1:(NumHFRefChannels+1)]  OutputSizes=1,1
  StftRef : Subsystem
  Spectra : Outport
  wires:
  StftRef/1(StftOut) -> Selector/1
  Matrix Concatenate/1 -> StftRef/1(data)
  Selector/1 -> Spectra/1
  RefIn/1 -> Matrix Concatenate/1
  MicIn/1 -> Matrix Concatenate/2
  Constant/1 -> Matrix Concatenate/3

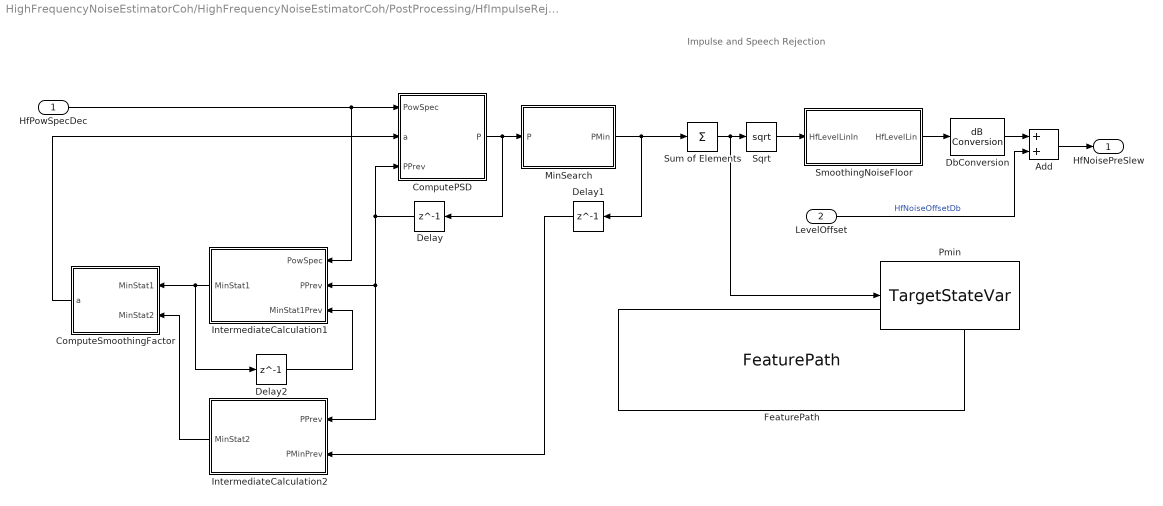
== system HighFrequencyNoiseEstimatorCoh/HighFrequencyNoiseEstimatorCoh/PostProcessing/HfImpulseRejection ==
  note: Impulse and Speech Rejection
  HfPowSpecDec : Inport
  LevelOffset : Inport  Port=2
  Add : Sum
  ComputePSD : Subsystem
  ComputeSmoothingFactor : Subsystem
  DbConversion : dspmathops/dB Conversion  dBtype=dB  intype=Amplitude  R=1  fuzz=on
  Delay : Delay  DelayLength=1  InitialCondition=0
  Delay1 : Delay  DelayLength=1  InitialCondition=1
  Delay2 : Delay  DelayLength=1  InitialCondition=0
  FeaturePath : FeaturePath/FeaturePath  FeatureName=ImpulseRejection  IsGroup=off  GroupNumber=-1  IsModule=off  TriggerInit=[750 304 1100 406]
      settings: SourceProductName=Bose Talaria
  "IntermediateCalculation1 " : Subsystem
  IntermediateCalculation2 : Subsystem
  MinSearch : Subsystem
  Pmin : StateVar/TargetStateVar  TriggerInit=[1015 256 1155 324]  TspName=Pmin  StateName=Pmin  UseSameName=on  IfdefMacro=[]
      settings: SourceProductName=Bose Talaria
  SmoothingNoiseFloor : Subsystem
  Sqrt : Sqrt
  Sum of Elements : Sum  Inputs=+
  HfNoisePreSlew : Outport  VectorParamsAs1DForOutWhenUnconnected=off
  wires:
  Add/1 -> HfNoisePreSlew/1
  DbConversion/1 -> Add/1
  SmoothingNoiseFloor/1(HfLevelLin) -> DbConversion/1
  Sum of Elements/1 -> Pmin/1, Sqrt/1
  Sqrt/1 -> SmoothingNoiseFloor/1(HfLevelLinIn)
  ComputeSmoothingFactor/1(a) -> ComputePSD/2(a)
  Delay1/1 -> IntermediateCalculation2/2(PMinPrev)
  IntermediateCalculation2/1(MinStat2) -> ComputeSmoothingFactor/2(MinStat2)
  Delay/1 -> ComputePSD/3(PPrev), IntermediateCalculation2/1(PPrev), "IntermediateCalculation1 "/2(PPrev)
  MinSearch/1(PMin) -> Sum of Elements/1, Delay1/1
  HfPowSpecDec/1 -> "IntermediateCalculation1 "/1(PowSpec), ComputePSD/1(PowSpec)
  ComputePSD/1(P) -> MinSearch/1(P), Delay/1
  Delay2/1 -> "IntermediateCalculation1 "/3(MinStat1Prev)
  "IntermediateCalculation1 "/1(MinStat1) -> Delay2/1, ComputeSmoothingFactor/1(MinStat1)
  LevelOffset/1 -> Add/2  "HfNoiseOffsetDb"

== system HighFrequencyNoiseEstimatorCoh/HighFrequencyNoiseEstimatorCoh/PostProcessing/HfSlew ==
  note: Slew for High-Frequency Noise Esimate
  HfNoisePreSlew : Inport  SampleTime=1/HFDecRate2
  Constant1 : Constant  Value=0  OutDataTypeStr=single
  Constant3 : Constant  Value=0  OutDataTypeStr=single
  FeaturePath : FeaturePath/FeaturePath  FeatureName=Slew  IsGroup=off  GroupNumber=-1  IsModule=off  TriggerInit=[85 39 200 146]
      settings: SourceProductName=Bose Talaria
  Slew : SpeedBoundsNoiseSlew/Slew  SystemSampleTime=-1  VariantActivationTime=update diagram  Latency=0  AutoFrameSizeCalculation=off
  attack : Subsystem
  decay : Subsystem
  init : Constant  Value=Config.SlewInitDb  OutDataTypeStr=single
  threshold : TuneVar/TuneTOP  TriggerInit=[30 282 255 318]  TopName=ThresholdDb  TuneName=ThresholdDb  DataType=single  TunabilityNumber=1  MinValue=[]  MaxValue=[]  BankNumber=0  PreOverlay=false  PostOverlay=false  UseSameName=on  MaskValue=Config.SlewThresholdDb
      settings: SourceProductName=Bose Talaria
  HfNoisePostSlew : Outport  VectorParamsAs1DForOutWhenUnconnected=off
  wires:
  Slew/1 -> HfNoisePostSlew/1
  HfNoisePreSlew/1 -> Slew/1
  Constant3/1 -> Slew/2
  decay/1(HfNoiseRefLatencySamples) -> Slew/4  "HfNoiseSlewDecayDbPerSample"
  attack/1(HfNoiseRefLatencySamples) -> Slew/3  "HfNoiseSlewAttackDbPerSample"
  threshold/1 -> Slew/5  "HfNoiseSlewThresholdDb"
  init/1 -> Slew/7  "HfNoiseSlewInitDb"
  Constant1/1 -> Slew/6

== system HighFrequencyNoiseEstimatorCoh/HighFrequencyNoiseEstimatorCoh/ReferenceLatency/RefLatency ==
  Captured Tune Const : TuneVar/CapturedTuneConst  TriggerInit=[-195 162 -95 198]  Role=Automatic
      settings: SourceProductName=Bose Talaria
  Constant : Constant  Value=Config.RefMaxLatencySamples  OutDataTypeStr=int32
  TOP : TOP/TOP  TriggerInit=[85 129 255 171]  TopName=RefLatencySamples  DataType=int32  BankNumber=0  PreOverlay=false  PostOverlay=false  Role=Automatic
      settings: SourceProductName=Bose Talaria
  TranslateTrigger : TuneVar/TranslateTrigger  TriggerInit=[-24 -20 14 35]
      settings: SourceProductName=Bose Talaria
  Tune Variable : TuneVar/TuneVar  TuneName=RefLatencyMs  SpecifyMaxSize=off  VariableDim=1 (Row)  MaxSize=[1 1]  TunabilityNumber=1  MinValue=[]  MaxValue=[]  TriggerInit=[-435 90 -240 140]  MaskValue=Config.RefLatencyMsec
      settings: SourceProductName=Bose Talaria
  ms2samples : MATLAB Function  TreatAsAtomicUnit=on
  hf_noise_ref_latency_samples : Outport  VectorParamsAs1DForOutWhenUnconnected=off
  wires:
  TranslateTrigger/1 -> ms2samples/Trigger
  Tune Variable/1 -> ms2samples/1(DelayTimeMS)  "RefLatencyMs"
  ms2samples/1(Samples) -> TOP/1
  TOP/1 -> hf_noise_ref_latency_samples/1  "RefLatencySamples"
  Constant/1 -> Captured Tune Const/1
  Captured Tune Const/1 -> ms2samples/2(MaxLatencySamples)

== system HighFrequencyNoiseEstimatorCoh/RatioCalculation/APLFUP/FlagHoldTime ==
  TOP : TOP/TOP  TriggerInit=[435 27 630 73]  TopName=FlagHoldTimeSamples  DataType=single  BankNumber=0  PreOverlay=false  PostOverlay=false  Role=Automatic
      settings: SourceProductName=Bose Talaria
  TranslateTrigger : TuneVar/TranslateTrigger  TriggerInit=[306 -100 344 -45]
      settings: SourceProductName=Bose Talaria
  Tune Variable : TuneVar/TuneVar  TuneName=FlagHoldTimeS  SpecifyMaxSize=off  VariableDim=1 (Row)  MaxSize=[1 1]  TunabilityNumber=1  MinValue=[]  MaxValue=[]  TriggerInit=[-35 27 160 73]  MaskValue=Config.UpdateFlagHoldTimeSec
      settings: SourceProductName=Bose Talaria
  sec2samples : MATLAB Function  TreatAsAtomicUnit=on
  Out1 : Outport  VectorParamsAs1DForOutWhenUnconnected=off
  wires:
  TOP/1 -> Out1/1  "FlagHoldTimeSamples"
  Tune Variable/1 -> sec2samples/1(time)  "FlagHoldTimeS"
  sec2samples/1(samples) -> TOP/1
  TranslateTrigger/1 -> sec2samples/Trigger

== system HighFrequencyNoiseEstimatorCoh/RatioCalculation/APLFUP/LfNoiseUpdatePeriod ==
  TOP : TOP/TOP  TriggerInit=[440 20 685 80]  TopName=LfNoiseUpdatePeriodSamples  DataType=single  BankNumber=0  PreOverlay=false  PostOverlay=false  Role=Automatic
      settings: SourceProductName=Bose Talaria
  TranslateTrigger : TuneVar/TranslateTrigger  TriggerInit=[306 -100 344 -45]
      settings: SourceProductName=Bose Talaria
  Tune Variable : TuneVar/TuneVar  TuneName=LfNoiseUpdatePeriodS  SpecifyMaxSize=off  VariableDim=1 (Row)  MaxSize=[1 1]  TunabilityNumber=1  MinValue=[]  MaxValue=[]  TriggerInit=[-100 20 145 80]  MaskValue=Config.UpdateLfNoiseUpdatePeriodSec
      settings: SourceProductName=Bose Talaria
  sec2samples : MATLAB Function  TreatAsAtomicUnit=on
  Out1 : Outport  VectorParamsAs1DForOutWhenUnconnected=off
  wires:
  TOP/1 -> Out1/1  "LfNoiseUpdatePeriodSamples"
  Tune Variable/1 -> sec2samples/1(time)  "LfNoiseUpdatePeriodS"
  sec2samples/1(samples) -> TOP/1
  TranslateTrigger/1 -> sec2samples/Trigger

== system HighFrequencyNoiseEstimatorCoh/RatioCalculation/RatioSlew/attack ==
  TOP : TOP/TOP  TriggerInit=[-10 87 195 133]  TopName=AttackDbPerSample  DataType=single  BankNumber=0  PreOverlay=false  PostOverlay=false  Role=Automatic
      settings: SourceProductName=Bose Talaria
  TranslateTrigger : TuneVar/TranslateTrigger  TriggerInit=[-119 -30 -81 25]
      settings: SourceProductName=Bose Talaria
  Tune Variable : TuneVar/TuneVar  TuneName=AttackDbPerS  SpecifyMaxSize=off  VariableDim=1 (Row)  MaxSize=[1 1]  TunabilityNumber=1  MinValue=[]  MaxValue=[]  TriggerInit=[-475 85 -305 135]  MaskValue=Config.SlewAttackDbpersec
      settings: SourceProductName=Bose Talaria
  sec2sample : MATLAB Function  TreatAsAtomicUnit=on
  Out1 : Outport  VectorParamsAs1DForOutWhenUnconnected=off
  wires:
  TOP/1 -> Out1/1  "AttackDbPerSample"
  sec2sample/1(y) -> TOP/1
  Tune Variable/1 -> sec2sample/1(u)  "AttackDbPerS"
  TranslateTrigger/1 -> sec2sample/Trigger

== system HighFrequencyNoiseEstimatorCoh/RatioCalculation/RatioSlew/decay ==
  TOP : TOP/TOP  TriggerInit=[-15 85 195 135]  TopName=DecayDbPerSample  DataType=single  BankNumber=0  PreOverlay=false  PostOverlay=false  Role=Automatic
      settings: SourceProductName=Bose Talaria
  TranslateTrigger : TuneVar/TranslateTrigger  TriggerInit=[-119 -30 -81 25]
      settings: SourceProductName=Bose Talaria
  Tune Variable : TuneVar/TuneVar  TuneName=DecayDbPerS  SpecifyMaxSize=off  VariableDim=1 (Row)  MaxSize=[1 1]  TunabilityNumber=1  MinValue=[]  MaxValue=[]  TriggerInit=[-485 85 -315 135]  MaskValue=Config.SlewDecayDbpersec
      settings: SourceProductName=Bose Talaria
  sec2sample : MATLAB Function  TreatAsAtomicUnit=on
  Out1 : Outport  VectorParamsAs1DForOutWhenUnconnected=off
  wires:
  TranslateTrigger/1 -> sec2sample/Trigger
  Tune Variable/1 -> sec2sample/1(u)  "DecayDbPerS"
  sec2sample/1(y) -> TOP/1
  TOP/1 -> Out1/1  "DecayDbPerSample"

== system HighFrequencyNoiseEstimatorCoh/RatioCalculation/RatioSmoother/InitUnDb ==
  " " : Inport
  Gain : Gain  Gain=0.05  SaturateOnIntegerOverflow=on  OutDataTypeStr=Inherit: Same as input  ParamDataTypeStr=Inherit: Same as input
  Math Function : Math  Operator=10^u  SignedPower=on
  "  " : Outport  VectorParamsAs1DForOutWhenUnconnected=off
  wires:
  " "/1 -> Gain/1
  Math Function/1 -> "  "/1
  Gain/1 -> Math Function/1

== system HighFrequencyNoiseEstimatorCoh/RatioCalculation/RatioSmoother/RatioImpulseRejectionGamma0 ==
  TOP : TOP/TOP  TriggerInit=[440 20 725 80]  TopName=Gamma0  DataType=single  BankNumber=0  PreOverlay=false  PostOverlay=false  Role=Automatic
      settings: SourceProductName=Bose Talaria
  Tau2Gamma : MATLAB Function  TreatAsAtomicUnit=on
  TranslateTrigger : TuneVar/TranslateTrigger  TriggerInit=[306 -100 344 -45]
      settings: SourceProductName=Bose Talaria
  Tune Variable : TuneVar/TuneVar  TuneName=Gamma0TauS  SpecifyMaxSize=off  VariableDim=1 (Row)  MaxSize=[1 1]  TunabilityNumber=1  MinValue=[]  MaxValue=[]  TriggerInit=[-195 25 60 75]  MaskValue=Config.ImpRejGamma0TauSec
      settings: SourceProductName=Bose Talaria
  Out1 : Outport  VectorParamsAs1DForOutWhenUnconnected=off
  wires:
  TOP/1 -> Out1/1  "Gamma0"
  Tune Variable/1 -> Tau2Gamma/1(tau)  "Gamma0TauS"
  Tau2Gamma/1(gamma) -> TOP/1
  TranslateTrigger/1 -> Tau2Gamma/Trigger

== system HighFrequencyNoiseEstimatorCoh/RatioCalculation/RatioSmoother/RatioImpulseRejectionImpulseVarianceLpfCoef ==
  TOP : TOP/TOP  TriggerInit=[285 19 540 81]  TopName=ImpulseVarianceLpfCoef  DataType=single  BankNumber=0  PreOverlay=false  PostOverlay=false  Role=Automatic
      settings: SourceProductName=Bose Talaria
  Tau2Coef : MATLAB Function  TreatAsAtomicUnit=on
  TranslateTrigger : TuneVar/TranslateTrigger  TriggerInit=[151 -115 189 -60]
      settings: SourceProductName=Bose Talaria
  Tune Variable : TuneVar/TuneVar  TuneName=ImpulseVarianceLpfTauS  SpecifyMaxSize=off  VariableDim=1 (Row)  MaxSize=[1 1]  TunabilityNumber=1  MinValue=[]  MaxValue=[]  TriggerInit=[-275 19 -20 81]  MaskValue=Config.ImpRejImpulseVarianceLpfTauSec
      settings: SourceProductName=Bose Talaria
  Out1 : Outport  VectorParamsAs1DForOutWhenUnconnected=off
  wires:
  TOP/1 -> Out1/1  "ImpulseVarianceLpfCoef"
  Tune Variable/1 -> Tau2Coef/1(tau)  "ImpulseVarianceLpfTauS"
  Tau2Coef/1(coef) -> TOP/1
  TranslateTrigger/1 -> Tau2Coef/Trigger

== system HighFrequencyNoiseEstimatorCoh/RatioCalculation/RatioSmoother/RatioUnDb ==
  " " : Inport
  Gain : Gain  Gain=0.05  SaturateOnIntegerOverflow=on  OutDataTypeStr=Inherit: Same as input  ParamDataTypeStr=Inherit: Same as input
  Math Function : Math  Operator=10^u  SignedPower=on
  "  " : Outport  VectorParamsAs1DForOutWhenUnconnected=off
  wires:
  Gain/1 -> Math Function/1
  Math Function/1 -> "  "/1
  " "/1 -> Gain/1

== system HighFrequencyNoiseEstimatorCoh/HighFrequencyNoiseEstimatorCoh/HfNoiseMusicSeparation /GaussianElimination/If Action Subsystem ==
  RefPowMin : Inport
  GXY : Inport  Port=2
  Action Port : ActionPort
  CoherenceModifier : MATLAB Function  TreatAsAtomicUnit=on
  Constant : Constant  Value=1.0  OutDataTypeStr=single
  FloorValue : MinMax  Function=max  Inputs=2
  GaussianElimination : MATLAB Function  TreatAsAtomicUnit=on
  Product1 : Product  RndMeth=Zero
  Subtract1 : Sum  Inputs=+-
  Out1 : Outport  VectorParamsAs1DForOutWhenUnconnected=off
  wires:
  Product1/1 -> FloorValue/1
  Constant/1 -> Subtract1/1
  GaussianElimination/1(c) -> CoherenceModifier/1("u ")
  RefPowMin/1 -> FloorValue/2
  CoherenceModifier/1(u) -> Subtract1/2
  GaussianElimination/2(Gyy) -> Product1/2
  Subtract1/1 -> Product1/1
  GXY/1 -> GaussianElimination/1(GXY)
  FloorValue/1 -> Out1/1

== system HighFrequencyNoiseEstimatorCoh/HighFrequencyNoiseEstimatorCoh/HfNoiseMusicSeparation /GaussianElimination/If Action Subsystem1 ==
  Gnn : Inport
  Action Port : ActionPort
  Out1 : Outport  VectorParamsAs1DForOutWhenUnconnected=off
  wires:
  Gnn/1 -> Out1/1

== system HighFrequencyNoiseEstimatorCoh/HighFrequencyNoiseEstimatorCoh/HfNoiseStft/EvenNumChannels/StftRef  ==
  data : Inport
  Buffer : Buffer  N=Config.CoherenceFftSize  V=Config.CoherenceOverlap
  RfftWindowing : RfftLib/RfftWindowing  Description=This block computes the Fourier Transform using an optimized FFT for real 2-channel input.  Config=Config.RfftWindowingStft
      settings: SourceProductName=Bose Blocklib
  const : Constant  Value=hamming(Config.CoherenceFftSize);  OutDataTypeStr=single
  StftOut : Outport  VectorParamsAs1DForOutWhenUnconnected=off
  wires:
  Buffer/1 -> RfftWindowing/1
  const/1 -> RfftWindowing/2
  data/1 -> Buffer/1
  RfftWindowing/1 -> StftOut/1

== system HighFrequencyNoiseEstimatorCoh/HighFrequencyNoiseEstimatorCoh/HfNoiseStft/OddNumChannels/StftRef ==
  data : Inport
  Buffer : Buffer  N=Config.CoherenceFftSize  V=Config.CoherenceOverlap
  RfftWindowing : RfftLib/RfftWindowing  Description=This block computes the Fourier Transform using an optimized FFT for real 2-channel input.  Config=Config.RfftWindowingStft
      settings: SourceProductName=Bose Blocklib
  const : Constant  Value=hamming(Config.CoherenceFftSize);  OutDataTypeStr=single
  StftOut : Outport  VectorParamsAs1DForOutWhenUnconnected=off
  wires:
  Buffer/1 -> RfftWindowing/1
  const/1 -> RfftWindowing/2
  data/1 -> Buffer/1
  RfftWindowing/1 -> StftOut/1

== system HighFrequencyNoiseEstimatorCoh/HighFrequencyNoiseEstimatorCoh/PostProcessing/HfImpulseRejection/ComputePSD ==
  PowSpec : Inport
  a : Inport  Port=2
  PPrev : Inport  Port=3
  Add : Sum
  Bias : Bias  Bias=1  SaturateOnIntegerOverflow=off
  Gain : Gain  Gain=-1
  Product : Product  RndMeth=Zero
  Product1 : Product  RndMeth=Zero
  P : Outport  VectorParamsAs1DForOutWhenUnconnected=off
  wires:
  Bias/1 -> Product/2
  Gain/1 -> Bias/1
  Add/1 -> P/1
  PPrev/1 -> Product1/2
  a/1 -> Gain/1, Product1/1
  PowSpec/1 -> Product/1
  Product/1 -> Add/1
  Product1/1 -> Add/2

== system HighFrequencyNoiseEstimatorCoh/HighFrequencyNoiseEstimatorCoh/PostProcessing/HfImpulseRejection/ComputeSmoothingFactor ==
  MinStat1 : Inport
  MinStat2 : Inport  Port=2
  Bias2 : Bias  Bias=eps  SaturateOnIntegerOverflow=off
  Divide : Product  Inputs=**/
  MinMax2 : MinMax  Function=max  Inputs=2
  MinstatAlphaFactor : TuneVar/TuneTOP  TriggerInit=[-230 62 145 98]  TopName=MinstatAlphaFactor  TuneName=MinstatAlphaFactor  DataType=single  TunabilityNumber=1  MinValue=[]  MaxValue=[]  BankNumber=0  PreOverlay=false  PostOverlay=false  UseSameName=on  MaskValue=Config.ImpRejMinStatAlphaFactor
      settings: SourceProductName=Bose Talaria
  MinstatAlphaMin : TuneVar/TuneTOP  TriggerInit=[-230 167 145 203]  TopName=MinstatAlphaMin  TuneName=MinstatAlphaMin  DataType=single  TunabilityNumber=1  MinValue=[]  MaxValue=[]  BankNumber=0  PreOverlay=false  PostOverlay=false  UseSameName=on  MaskValue=Config.ImpRejMinStatAlphaMin
      settings: SourceProductName=Bose Talaria
  a : Outport  VectorParamsAs1DForOutWhenUnconnected=off
  wires:
  Bias2/1 -> Divide/3
  MinMax2/1 -> a/1
  MinStat2/1 -> Bias2/1
  MinStat1/1 -> Divide/2
  Divide/1 -> MinMax2/1
  MinstatAlphaFactor/1 -> Divide/1  "HfNoiseImpulseRejectionMinstatAlphaFactor"
  MinstatAlphaMin/1 -> MinMax2/2  "HfNoiseImpulseRejectionMinstatAlphaMin"

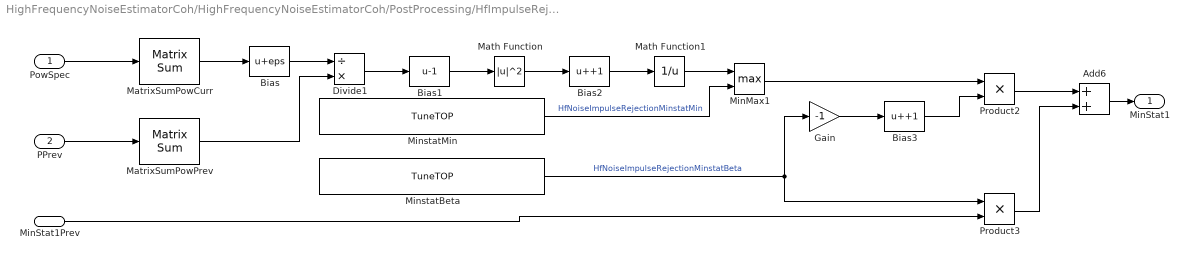
== system HighFrequencyNoiseEstimatorCoh/HighFrequencyNoiseEstimatorCoh/PostProcessing/HfImpulseRejection/IntermediateCalculation1  ==
  PowSpec : Inport
  PPrev : Inport  Port=2
  MinStat1Prev : Inport  Port=3
  Add6 : Sum
  Bias : Bias  Bias=eps  SaturateOnIntegerOverflow=off
  Bias1 : Bias  Bias=-1  SaturateOnIntegerOverflow=off
  Bias2 : Bias  Bias=+1  SaturateOnIntegerOverflow=off
  Bias3 : Bias  Bias=+1  SaturateOnIntegerOverflow=off
  Divide1 : Product  Inputs=/*
  Gain : Gain  Gain=-1
  Math Function : Math  Operator=magnitude^2  SignedPower=on
  Math Function1 : Math  Operator=reciprocal  SignedPower=on
  MatrixSumPowCurr : dspobslib/Matrix Sum  Dim=Columns  roundingMode=Floor  overflowMode=off
  MatrixSumPowPrev : dspobslib/Matrix Sum  Dim=Columns  roundingMode=Floor  overflowMode=off
  MinMax1 : MinMax  Function=max  Inputs=2
  MinstatBeta : TuneVar/TuneTOP  TriggerInit=[310 147 535 183]  TopName=MinstatBeta  TuneName=MinstatBeta  DataType=single  TunabilityNumber=1  MinValue=[]  MaxValue=[]  BankNumber=0  PreOverlay=false  PostOverlay=false  UseSameName=on  MaskValue=Config.ImpRejMinStatBeta
      settings: SourceProductName=Bose Talaria
  MinstatMin : TuneVar/TuneTOP  TriggerInit=[310 87 535 123]  TopName=MinstatMin  TuneName=MinstatMin  DataType=single  TunabilityNumber=1  MinValue=[]  MaxValue=[]  BankNumber=0  PreOverlay=false  PostOverlay=false  UseSameName=on  MaskValue=Config.ImpRejMinStatMin
      settings: SourceProductName=Bose Talaria
  Product2 : Product  RndMeth=Zero
  Product3 : Product  RndMeth=Zero
  MinStat1 : Outport  VectorParamsAs1DForOutWhenUnconnected=off
  wires:
  Gain/1 -> Bias3/1
  MinStat1Prev/1 -> Product3/2
  Add6/1 -> MinStat1/1
  PPrev/1 -> MatrixSumPowPrev/1
  PowSpec/1 -> MatrixSumPowCurr/1
  MatrixSumPowCurr/1 -> Bias/1
  MatrixSumPowPrev/1 -> Divide1/2
  Divide1/1 -> Bias1/1
  Bias1/1 -> Math Function/1
  Math Function/1 -> Bias2/1
  Bias2/1 -> Math Function1/1
  Math Function1/1 -> MinMax1/1
  MinMax1/1 -> Product2/1
  Bias/1 -> Divide1/1
  Bias3/1 -> Product2/2
  Product2/1 -> Add6/1
  Product3/1 -> Add6/2
  MinstatMin/1 -> MinMax1/2  "HfNoiseImpulseRejectionMinstatMin"
  MinstatBeta/1 -> Gain/1, Product3/1  "HfNoiseImpulseRejectionMinstatBeta"

== system HighFrequencyNoiseEstimatorCoh/HighFrequencyNoiseEstimatorCoh/PostProcessing/HfImpulseRejection/IntermediateCalculation2 ==
  PPrev : Inport
  PMinPrev : Inport  Port=2
  Bias : Bias  Bias=eps  SaturateOnIntegerOverflow=off
  Bias1 : Bias  Bias=-1  SaturateOnIntegerOverflow=off
  Bias2 : Bias  Bias=+1  SaturateOnIntegerOverflow=off
  Divide2 : Product  Inputs=*/
  Math Function2 : Math  Operator=magnitude^2  SignedPower=on
  MinStat2 : Outport  VectorParamsAs1DForOutWhenUnconnected=off
  wires:
  Bias2/1 -> MinStat2/1
  PMinPrev/1 -> Bias/1
  PPrev/1 -> Divide2/1
  Divide2/1 -> Bias1/1
  Bias1/1 -> Math Function2/1
  Math Function2/1 -> Bias2/1
  Bias/1 -> Divide2/2
